simulink model "battery12VwithBattery"  (R2019a)
settings: Solver=ode45  StartTime=0.0  StopTime=2  RelTol=1e-3  EnableMultiTasking=on
undefined symbols (not defined in the file or in its folder): Acid, Lead
libraries: powerlib x10, simulink x2, electricdrivelib x1, powerlib_meascontrol x1
settings Model: Creator=Tushar  LastModifiedBy=stushar
settings DataIOCC: LimitDataPoints=on  SaveFormat=Array  ReturnWorkspaceOutputs=off
settings OptimizationCC: LifeSpan=inf
settings DebuggingCC: SFUnexpectedBacktrackingDiag=warning  SFNoUnconditionalDefaultTransitionDiag=warning  SFExecutionAtInitializationDiag=none  ArithmeticOperatorsInVariantConditions=warning
settings HardwareCC: ProdBitPerPointer=32  ProdBitPerSizeT=32  ProdBitPerPtrDiffT=32  ProdLargestAtomicFloat=None  ProdIntDivRoundTo=Undefined  ProdEndianess=Unspecified  ProdWordSize=32  ProdHWDeviceType=32-bit Generic
settings ModelReferenceCC: PropagateSignalLabelsOutOfModel=off
settings SFSimCC: SimUseLocalCustomCode=off
settings RTWCC: RTWUseLocalCustomCode=off
settings CodeAppCC: StateflowObjectComments=on
settings GRTTargetCC: TargetLangStandard=C89/C90 (ANSI)  GeneratePreprocessorConditionals=Disable all
settings ConfigComp: CovMetricSettings=dw  CovHtmlReporting=on  CovSaveCumulativeToWorkspaceVar=on  CovSaveSingleToWorkspaceVar=on  CovExternalEMLEnable=off
settings SimscapeCC: SimscapeNormalizeSystem=off

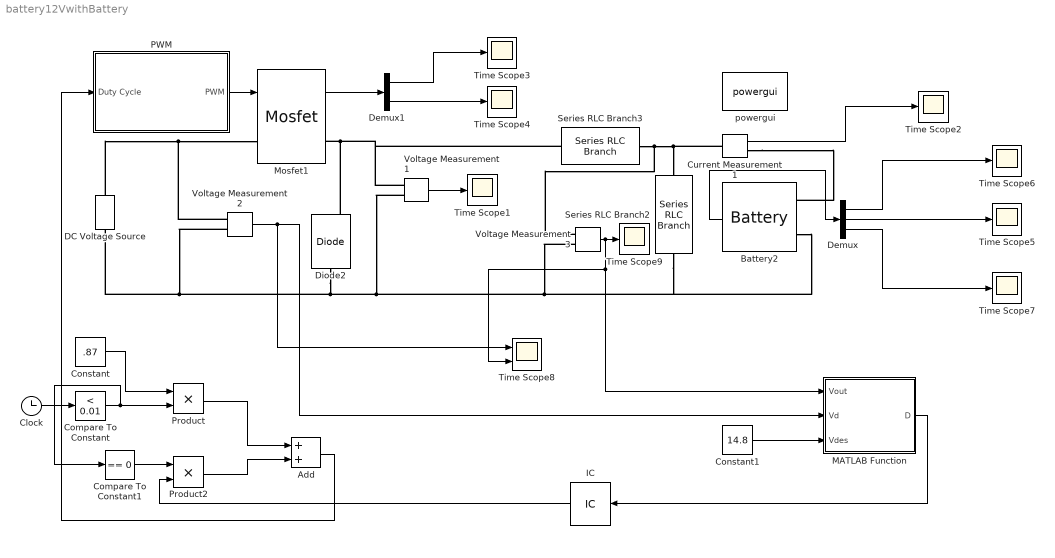
== system battery12VwithBattery ==
  Add : Sum
  Battery2 : electricdrivelib/Extra Sources/Battery  BatType=Lead-Acid  ShowTempParam=off  ThermalPreset=no  ShowAgeParam=off  NomV=12  NomQ=18  SOC=0  Batt_Tr=10e-6  PresetModel=on  MaxQ=18.75  MinV=9  FullV=13.0658  Dis_rate=3.6  R=0.0066667  Normal_OP=5.585  expZone="[12.2171         0.06]"  current=[6.5 13 32.5]  Units=Time  Tci=20  NomT=20  T2=-30  MaxQ2=4.8  FullV2=7.1  Normal_OP2=5.655  expZone2="[6.58           1]"  Rca=0.6  ti=2000  Dp=0  Neq0=0  Tsim=1e6  Ta1=25  Qeol=5.4*0.9  Reol=0.013333*1.2  Char_age=[2.3478, 3]  Dis_age=[2.3478, 10]  N1=1500  N2=10500  N3=1000  N4=1400  Ta2=45  N5=950
      settings: SourceProductName=Simscape Electrical
  Clock : Clock
  Compare To Constant : simulink/Logic and Bit Operations/Compare To Constant  relop=<  const=0.01  OutDataTypeStr=boolean
  Compare To Constant1 : simulink/Logic and Bit Operations/Compare To Constant  relop===  const=0  OutDataTypeStr=boolean
  Constant : Constant  Value=.87
  Constant1 : Constant  Value=14.8
  Current Measurement1 : powerlib/Measurements/Current Measurement  PhasorSimulation=off  OutputType=Complex  PSBequivalent=0
      settings: SourceProductName=Simscape Electrical
  DC Voltage Source : powerlib/Electrical Sources/DC Voltage Source  Amplitude=22  Measurements=Voltage
      settings: SourceProductName=Simscape Electrical
  Demux : Demux  Outputs=3
  Demux1 : Demux  Outputs=2
  Diode2 : powerlib/Power Electronics/Diode  Ron=0.00001  Lon=0  Vf=0  IC=0  UseSnubber=off  Rs=500  Cs=250e-9  Measurements=on
      settings: SourceProductName=Simscape Electrical
  IC : InitialCondition
  MATLAB Function : MATLAB Function  TreatAsAtomicUnit=on
  Mosfet1 : powerlib/Power Electronics/Mosfet  Ron=0.0001  Lon=0  Rd=0.001  Vfd=0  IC=0  Rs=42  Cs=600e-12  Measurements=on
      settings: SourceProductName=Simscape Electrical
  PWM : Subsystem
  Product : Product
  Product2 : Product
  Series RLC Branch2 : powerlib/Elements/Series RLC Branch  LConnTagsString=__new0  RConnTagsString=__new0  BranchType=RC  Resistance=.0015  Inductance=1e-3  SetiL0=off  InitialCurrent=0  Capacitance=100e-6  Setx0=on  InitialVoltage=0  Measurements=Branch voltage
      settings: SourceProductName=Simscape Electrical
  Series RLC Branch3 : powerlib/Elements/Series RLC Branch  LConnTagsString=__new0  RConnTagsString=__new0  BranchType=RL  Resistance=1.4e-3  Inductance=420e-6  SetiL0=off  InitialCurrent=0  Capacitance=1e-6  Setx0=off  InitialVoltage=0  Measurements=None
      settings: SourceProductName=Simscape Electrical
  Time Scope{1..7,9} (8 alike) : Scope
  Time Scope8 : Scope  NumInputPorts=2
  Voltage Measurement1 : powerlib/Measurements/Voltage Measurement  PhasorSimulation=off  OutputType=Complex  PSBequivalent=0
      settings: SourceProductName=Simscape Electrical
  Voltage Measurement2 : powerlib/Measurements/Voltage Measurement  PhasorSimulation=off  OutputType=Complex  PSBequivalent=0
      settings: SourceProductName=Simscape Electrical
  Voltage Measurement3 : powerlib/Measurements/Voltage Measurement  PhasorSimulation=off  OutputType=Complex  PSBequivalent=0
      settings: SourceProductName=Simscape Electrical
  powergui : powerlib/powergui  Priority=1  SimulationMode=Discrete  SampleTime=10e-7  frequency=60  Iterations=50  frequencyindice=0  Pbase=100e6  ErrMax=1e-4  UnitsV=kV  UnitsW=MW  buscounter=0  FunctionMessages=off  echomessages=off  EnableUseOfTLC=off  CurrentSourceSwitches=off  DisableSnubberDevices=off  DisableRonSwitches=off  DisableVfSwitches=off  DisplayEquations=off  AutomaticDiscreteSolvers=off  SolverType=Tustin/Backward Euler (TBE)  Interpol=off  ExternalGateDelay=off  methode=off  Ts=100  x0status=blocks  SPID=off  SwTol=0  HookPort=off  NonlinearTolerance=0  nMaxIteration=15  ContinueOnMaxIteration=off  RestoreLinks=warning  ResistiveCurrentMeasurement=off  Frange=[0:2:500]  Ylog=off  Xlog=on  ShowGrid=off  save=off  variable=ZData  structure=0  ZoomFFT=off  StartTime=0.0  cycles=1  DisplayStyle=1  fundamental=60  FreqAxis=off  MaxFrequency=1000  frequencyindicesteady=1  RmsSteady=1  display=off
      settings: SourceProductName=Simscape Electrical
  wires:
  PWM/1(PWM) -> Mosfet1/1
  Current Measurement1/1 -> Time Scope2/1
  Voltage Measurement3/1 -> Time Scope8/2, MATLAB Function/1(Vout), Time Scope9/1
  Voltage Measurement1/1 -> Time Scope1/1
  Battery2/1 -> Demux/1
  Demux/1 -> Time Scope6/1
  Demux/2 -> Time Scope5/1
  Demux/3 -> Time Scope7/1
  Voltage Measurement2/1 -> Time Scope8/1, MATLAB Function/2(Vd)
  Constant1/1 -> MATLAB Function/3(Vdes)
  Clock/1 -> Compare To Constant/1
  Constant/1 -> Product/1
  Compare To Constant/1 -> Compare To Constant1/1, Product/2
  Compare To Constant1/1 -> Product2/1
  Product/1 -> Add/1
  Product2/1 -> Add/2
  Add/1 -> PWM/1("Duty Cycle ")
  IC/1 -> Product2/2
  MATLAB Function/1(D) -> IC/1
  Mosfet1/1 -> Demux1/1
  Demux1/1 -> Time Scope3/1
  Demux1/2 -> Time Scope4/1
  connections:
  Voltage Measurement3/LConn1 -- Series RLC Branch3/RConn1 -- Series RLC Branch2/LConn1 -- Current Measurement1/LConn1
  Mosfet1/RConn1 -- Voltage Measurement1/LConn1 -- Series RLC Branch3/LConn1 -- Diode2/RConn1
  Voltage Measurement1/LConn2 -- Voltage Measurement3/LConn2 -- Series RLC Branch2/RConn1 -- Battery2/LConn2 -- Diode2/LConn1 -- Voltage Measurement2/LConn2 -- DC Voltage Source/LConn1
  DC Voltage Source/RConn1 -- Voltage Measurement2/LConn1 -- Mosfet1/LConn1
  Current Measurement1/RConn1 -- Battery2/LConn1

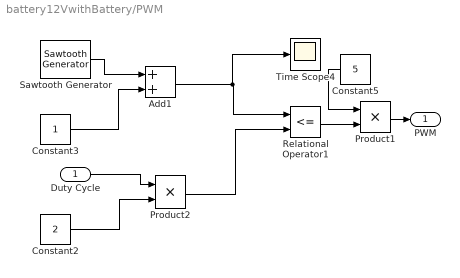
== system battery12VwithBattery/PWM ==
  "Duty Cycle " : Inport
  Add1 : Sum
  Constant2 : Constant  Value=2
  Constant3 : Constant
  Constant5 : Constant  Value=5
  Product1 : Product
  Product2 : Product
  Relational Operator1 : RelationalOperator  Operator=<=  OutDataTypeStr=boolean  RndMeth=Nearest
  Sawtooth Generator : powerlib_meascontrol/Pulse & Signal Generators/Sawtooth Generator  Freq=40000  Phase=0  Ts=0
      settings: SourceProductName=Simscape Electrical
  Time Scope4 : Scope
  PWM : Outport
  wires:
  Relational Operator1/1 -> Product1/2
  Product2/1 -> Relational Operator1/2
  Sawtooth Generator/1 -> Add1/1
  Constant5/1 -> Product1/1
  Constant3/1 -> Add1/2
  Add1/1 -> Time Scope4/1, Relational Operator1/1
  Product1/1 -> PWM/1
  "Duty Cycle "/1 -> Product2/1
  Constant2/1 -> Product2/2

== matlab function battery12VwithBattery/MATLAB Function ==
  data: Vout input; D output; Vd input; Vdes input
function D = fcn(Vout,Vd,Vdes)
Dgiven=Vdes/Vd;
Dfound=Vout/Vd;
%#codegen
Derror=(Dgiven-Dfound)/Dgiven;
D=Dgiven/(1-Derror);
